simulink model "func1"  (R2016b)
settings: Solver=VariableStepAuto  StartTime=0.0  StopTime=10.0  RelTol=1e-3
settings Model: Creator=Ashraf  LastModifiedBy=Ashraf

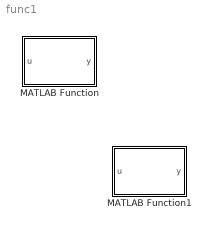
== system func1 ==
  MATLAB Function : MATLAB Function  TreatAsAtomicUnit=on
  MATLAB Function1 : MATLAB Function  TreatAsAtomicUnit=on

== matlab function func1/MATLAB Function1 ==
  data: u input; y output
function y = fcn(u)

y = u;

== matlab function func1/MATLAB Function ==
  data: u input; y output
function y = fcn(u)
y=sum(u);
